simulink model "mars_uav_simulink"  (R2021a)
settings: Solver=ode45  StartTime=0.0  StopTime=30  RelTol=1e-3  EnableMultiTasking=on
undefined symbols (not defined in the file or in its folder): Quad, sigbuilder_block
settings Model: Creator=test  LastModifiedBy=aakash
settings SolverCC: AlgebraicLoopSolver=TrustRegion
settings DataIOCC: SaveFormat=Array  SignalLoggingSaveFormat=ModelDataLogs  ReturnWorkspaceOutputs=off
settings OptimizationCC: ExpressionDepthLimit=2147483647  LifeSpan=inf
settings DebuggingCC: UnderspecifiedInitializationDetection=Classic  MergeDetectMultiDrivingBlocksExec=none  SolverPrmCheckMsg=warning  FcnCallInpInsideContextMsg=warning  StateNameClashWarn=warning  SFUnexpectedBacktrackingDiag=warning  SFNoUnconditionalDefaultTransitionDiag=warning  SFExecutionAtInitializationDiag=none  SFMachineParentedDataDiag=warning  ArithmeticOperatorsInVariantConditions=warning
settings HardwareCC: ProdBitPerPointer=32  ProdBitPerSizeT=32  ProdBitPerPtrDiffT=32  ProdLargestAtomicFloat=None  ProdIntDivRoundTo=Undefined  ProdEndianess=Unspecified  ProdWordSize=32  ProdHWDeviceType=32-bit Generic
settings ModelReferenceCC: PropagateSignalLabelsOutOfModel=off
settings SFSimCC: SimUseLocalCustomCode=off  CustomCodeUndefinedFunction=UseInterfaceOnly
settings RTWCC: RTWUseLocalCustomCode=off
settings CodeAppCC: StateflowObjectComments=on
settings GRTTargetCC: TargetLangStandard=C89/C90 (ANSI)  CombineOutputUpdateFcns=off  GRTInterface=on
settings ConfigComp: CovMetricSettings=dw  CovSaveCumulativeToWorkspaceVar=on  CovSaveSingleToWorkspaceVar=on

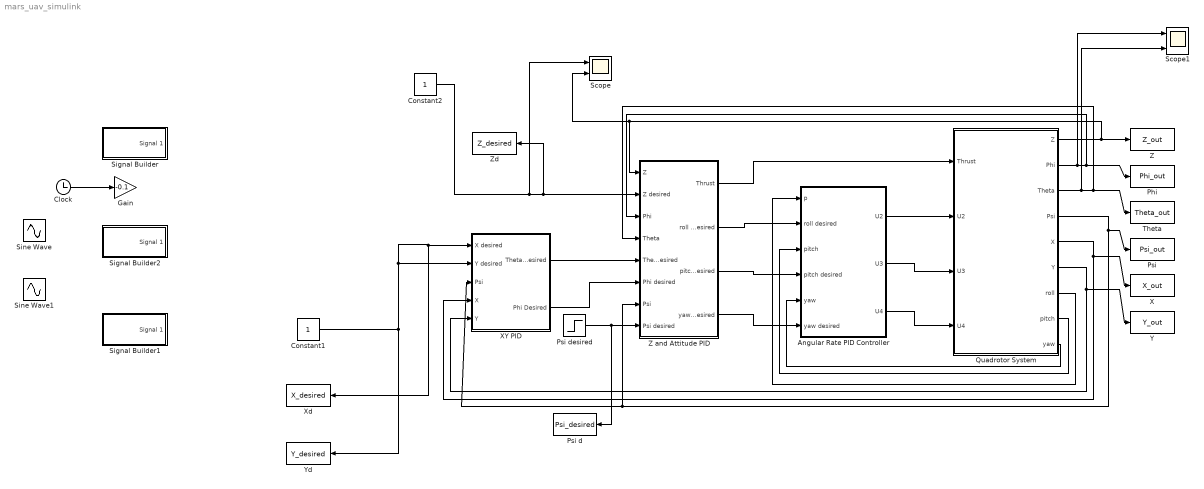
== system mars_uav_simulink ==
  Angular Rate PID Controller : Subsystem
  Clock : Clock
  Constant1 : Constant
  Constant2 : Constant
  Gain : Gain  Gain=-0.1
  Phi : ToWorkspace  VariableName=Phi_out  SaveFormat=Structure  SampleTime=-1
  Psi : ToWorkspace  VariableName=Psi_out  SaveFormat=Structure  SampleTime=-1
  Psi d : ToWorkspace  VariableName=Psi_desired  SaveFormat=Structure  SampleTime=-1
  Psi desired : Step  After=0  SampleTime=0
  Quadrotor System : Subsystem
  Scope : Scope  NumInputPorts=2
  Scope1 : Scope  NumInputPorts=2
  Signal Builder : Subsystem  Tag=STV Subsys  LoadFcn=sigbuilder_block('load');  StartFcn=sigbuilder_block('start');  StopFcn=sigbuilder_block('stop');  ClipboardFcn=sigbuilder_block('clipboard');  mask(Sigbuilder block){tuvar=[0:10]}
      mask help: Simulink:masks:SigbuilderBlock_MD
      mask init:
      | if ~strcmp(get_param(bdroot(gcbh),'SimulationStatus'),'stopped') tuvar = sigbuilder_block('maskInit'); end
      settings: CopyFcn=sigbuilder_block('copy');  DeleteFcn=sigbuilder_block('delete');  ModelCloseFcn=sigbuilder_block('modelClose');  PreSaveFcn=sigbuilder_block('preSave');  PauseFcn=sigbuilder_block('pause');  ContinueFcn=sigbuilder_block('continue');  NameChangeFcn=sigbuilder_block('namechange');  OpenFcn=sigbuilder_block('open',[437.6 199.2 550.4 400 ]);  CloseFcn=sigbuilder_block('close');
      mask Display: plot(0, 0, 100, 100,[2, 2, 32, 32, 2], [68, 8, 8, 68, 68],[32, 2], [38, 38], [32, 19, 2],[53, 60, 44], [32, 17, 17, 2],[16, 16, 31, 31]);txt = getActiveGroup(gcbh);text(2, 100, txt,'verticalAlignment', 'top');
  Signal Builder1 : Subsystem  Tag=STV Subsys  LoadFcn=sigbuilder_block('load');  StartFcn=sigbuilder_block('start');  StopFcn=sigbuilder_block('stop');  ClipboardFcn=sigbuilder_block('clipboard');  mask(Sigbuilder block){tuvar=[0:10]}
      mask help: Simulink:masks:SigbuilderBlock_MD
      mask init:
      | if ~strcmp(get_param(bdroot(gcbh),'SimulationStatus'),'stopped') tuvar = sigbuilder_block('maskInit'); end
      settings: CopyFcn=sigbuilder_block('copy');  DeleteFcn=sigbuilder_block('delete');  ModelCloseFcn=sigbuilder_block('modelClose');  PreSaveFcn=sigbuilder_block('preSave');  PauseFcn=sigbuilder_block('pause');  ContinueFcn=sigbuilder_block('continue');  NameChangeFcn=sigbuilder_block('namechange');  OpenFcn=sigbuilder_block('open',[437.6 199.2 550.4 400 ]);  CloseFcn=sigbuilder_block('close');
      mask Display: plot(0, 0, 100, 100,[2, 2, 32, 32, 2], [68, 8, 8, 68, 68],[32, 2], [38, 38], [32, 19, 2],[53, 60, 44], [32, 17, 17, 2],[16, 16, 31, 31]);txt = getActiveGroup(gcbh);text(2, 100, txt,'verticalAlignment', 'top');
  Signal Builder2 : Subsystem  Tag=STV Subsys  LoadFcn=sigbuilder_block('load');  StartFcn=sigbuilder_block('start');  StopFcn=sigbuilder_block('stop');  ClipboardFcn=sigbuilder_block('clipboard');  mask(Sigbuilder block){tuvar=[0:10]}
      mask help: Simulink:masks:SigbuilderBlock_MD
      mask init:
      | if ~strcmp(get_param(bdroot(gcbh),'SimulationStatus'),'stopped') tuvar = sigbuilder_block('maskInit'); end
      settings: CopyFcn=sigbuilder_block('copy');  DeleteFcn=sigbuilder_block('delete');  ModelCloseFcn=sigbuilder_block('modelClose');  PreSaveFcn=sigbuilder_block('preSave');  PauseFcn=sigbuilder_block('pause');  ContinueFcn=sigbuilder_block('continue');  NameChangeFcn=sigbuilder_block('namechange');  OpenFcn=sigbuilder_block('open',[437.6 199.2 550.4 400 ]);  CloseFcn=sigbuilder_block('close');
      mask Display: plot(0, 0, 100, 100,[2, 2, 32, 32, 2], [68, 8, 8, 68, 68],[32, 2], [38, 38], [32, 19, 2],[53, 60, 44], [32, 17, 17, 2],[16, 16, 31, 31]);txt = getActiveGroup(gcbh);text(2, 100, txt,'verticalAlignment', 'top');
  Sine Wave : Sin  Bias=-1  Frequency=0.1*pi  Phase=pi/2  SampleTime=0
  Sine Wave1 : Sin  Frequency=0.1*pi  SampleTime=0
  Theta : ToWorkspace  VariableName=Theta_out  SaveFormat=Structure  SampleTime=-1
  X : ToWorkspace  VariableName=X_out  SaveFormat=Structure  SampleTime=-1
  XY PID : Subsystem
  Xd : ToWorkspace  VariableName=X_desired  SaveFormat=Structure  SampleTime=-1
  Y : ToWorkspace  VariableName=Y_out  SaveFormat=Structure  SampleTime=-1
  Yd : ToWorkspace  VariableName=Y_desired  SaveFormat=Structure  SampleTime=-1
  Z : ToWorkspace  VariableName=Z_out  SaveFormat=Structure  SampleTime=-1
  Z and Attitude PID : Subsystem
  Zd : ToWorkspace  VariableName=Z_desired  SaveFormat=Structure  SampleTime=-1
  wires:
  Quadrotor System/2(Phi) -> Scope1/1, Phi/1, Z and Attitude PID/3(Phi)
  Quadrotor System/3(Theta) -> Scope1/2, Z and Attitude PID/4(Theta), Theta/1
  Quadrotor System/4(Psi) -> Psi/1, XY PID/3(Psi), Z and Attitude PID/7(Psi)
  Quadrotor System/5(X) -> X/1, XY PID/4(X)
  Quadrotor System/6(Y) -> Y/1, XY PID/5(Y)
  Quadrotor System/1(Z) -> Scope/2, Z and Attitude PID/1(Z), Z/1
  Psi desired/1 -> Z and Attitude PID/8(Psi desired), Psi d/1
  Constant1/1 -> XY PID/1(X desired), Xd/1, XY PID/2(Y desired), Yd/1
  Z and Attitude PID/1(Thrust) -> Quadrotor System/1(Thrust)
  XY PID/2(Phi Desired) -> Z and Attitude PID/6(Phi desired)
  Z and Attitude PID/2(roll desired) -> Angular Rate PID Controller/2(roll desired)
  Z and Attitude PID/3(pitch desired) -> Angular Rate PID Controller/4(pitch desired)
  Z and Attitude PID/4(yaw desired) -> Angular Rate PID Controller/6(yaw desired)
  Quadrotor System/9(yaw) -> Angular Rate PID Controller/5(yaw)
  Quadrotor System/8(pitch) -> Angular Rate PID Controller/3(pitch)
  Quadrotor System/7(roll) -> Angular Rate PID Controller/1(p)
  Angular Rate PID Controller/3(U4) -> Quadrotor System/4(U4)
  Angular Rate PID Controller/2(U3) -> Quadrotor System/3(U3)
  Angular Rate PID Controller/1(U2) -> Quadrotor System/2(U2)
  Clock/1 -> Gain/1
  XY PID/1(Theta Desired) -> Z and Attitude PID/5(Theta desired)
  Constant2/1 -> Scope/1, Zd/1, Z and Attitude PID/2(Z desired)

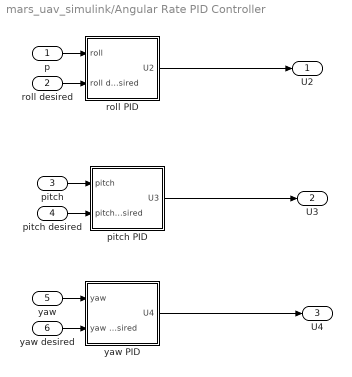
== system mars_uav_simulink/Angular Rate PID Controller ==
  p : Inport
  roll desired : Inport  Port=2
  pitch : Inport  Port=3
  pitch desired : Inport  Port=4
  yaw : Inport  Port=5
  yaw desired : Inport  Port=6
  pitch PID : Subsystem
  roll PID : Subsystem
  yaw PID : Subsystem
  U2 : Outport
  U3 : Outport  Port=2
  U4 : Outport  Port=3
  wires:
  roll PID/1(U2) -> U2/1
  pitch PID/1(U3) -> U3/1
  yaw PID/1(U4) -> U4/1
  p/1 -> roll PID/1(roll)
  roll desired/1 -> roll PID/2(roll desired)
  pitch/1 -> pitch PID/1(pitch)
  pitch desired/1 -> pitch PID/2(pitch desired)
  yaw/1 -> yaw PID/1(yaw)
  yaw desired/1 -> yaw PID/2(yaw desired)

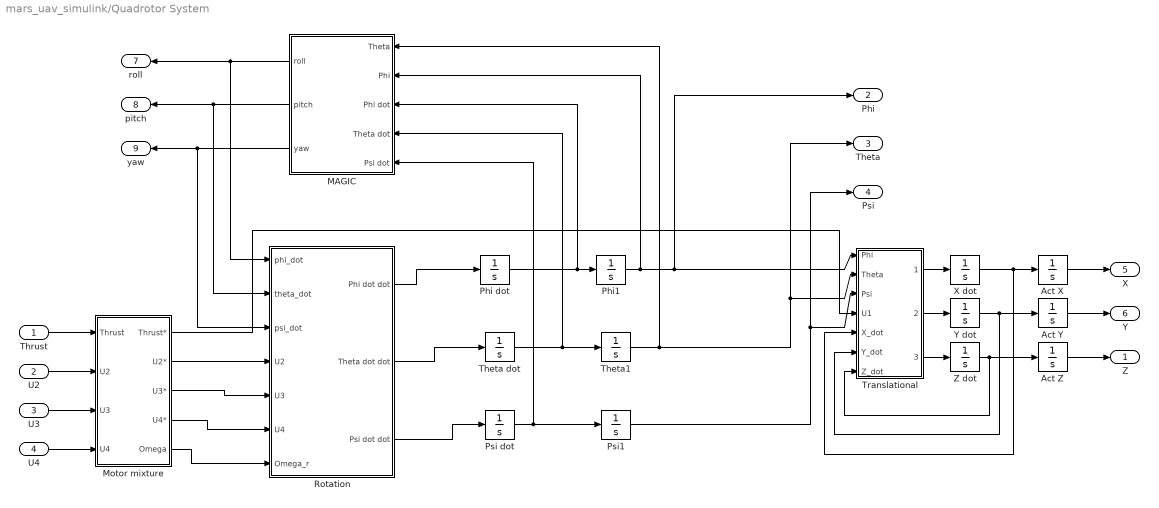
== system mars_uav_simulink/Quadrotor System ==
  Thrust : Inport
  U2 : Inport  Port=2
  U3 : Inport  Port=3
  U4 : Inport  Port=4
  Act X : Integrator
  Act Y : Integrator
  Act Z : Integrator
  "MAGIC " : Subsystem
  Motor mixture : Subsystem
  Phi dot : Integrator
  Phi1 : Integrator  ZeroCross=off
  Psi dot : Integrator  ZeroCross=off
  Psi1 : Integrator  ZeroCross=off
  "Rotation " : Subsystem
  Theta dot : Integrator  ZeroCross=off
  Theta1 : Integrator  ZeroCross=off
  Translational : Subsystem
  X dot : Integrator
  Y dot : Integrator
  Z dot : Integrator
  Z : Outport
  Phi : Outport  Port=2
  Theta : Outport  Port=3
  Psi : Outport  Port=4
  X : Outport  Port=5
  Y : Outport  Port=6
  roll : Outport  Port=7
  pitch : Outport  Port=8
  yaw : Outport  Port=9
  wires:
  "Rotation "/2(Theta dot dot) -> Theta dot/1
  Motor mixture/5(Omega) -> "Rotation "/7(Omega_r)
  Phi1/1 -> Translational/1(Phi), Phi/1, "MAGIC "/2(Phi)
  Theta1/1 -> Translational/2(Theta), Theta/1, "MAGIC "/1(Theta)
  Psi1/1 -> Translational/3(Psi), Psi/1
  Translational/1(X_dot_dot) -> X dot/1
  X dot/1 -> Act X/1, Translational/5(X_dot)
  Y dot/1 -> Act Y/1, Translational/6(Y_dot)
  Translational/2(Y_dot_dot) -> Y dot/1
  Z dot/1 -> Translational/7(Z_dot), Act Z/1
  Translational/3(Z_dot_dot) -> Z dot/1
  Act X/1 -> X/1
  Act Y/1 -> Y/1
  Act Z/1 -> Z/1
  Psi dot/1 -> Psi1/1, "MAGIC "/5(Psi dot)
  Theta dot/1 -> Theta1/1, "MAGIC "/4(Theta dot)
  Phi dot/1 -> Phi1/1, "MAGIC "/3(Phi dot)
  "Rotation "/3(Psi dot dot) -> Psi dot/1
  "Rotation "/1(Phi dot dot) -> Phi dot/1
  U4/1 -> Motor mixture/4(U4)
  U2/1 -> Motor mixture/2(U2)
  U3/1 -> Motor mixture/3(U3)
  Motor mixture/2(U2*) -> "Rotation "/4(U2)
  Motor mixture/3(U3*) -> "Rotation "/5(U3)
  Motor mixture/1(Thrust*) -> Translational/4(U1)
  Motor mixture/4(U4*) -> "Rotation "/6(U4)
  "MAGIC "/1(roll) -> roll/1, "Rotation "/1(phi_dot)
  "MAGIC "/2(pitch) -> pitch/1, "Rotation "/2(theta_dot)
  "MAGIC "/3(yaw) -> yaw/1, "Rotation "/3(psi_dot)
  Thrust/1 -> Motor mixture/1(Thrust)

== system mars_uav_simulink/Signal Builder ==
  Demux : Demux  Tag=STV Demux  Outputs=1
      settings: DisplayOption=none
  FromWs : FromWorkspace  Tag=STV FromWs  VariableName=tuvar
      SigBuilderData=|
      | common.afterFinalStr = 'Extrapolate'
      | common.sampleTime = 0
      | dataSet.timeRange = [0 30]
      | dataSet.name = 'Group 1'
      | sbobj.Groups.Name = 'Group 1'
      | sbobj.Groups.Signals.Name = 'Signal 1'
      | sbobj.Groups.Signals.XData = [0 5 10 20 25 30]
      | sbobj.Groups.Signals.YData = [0 1 1 -1 -1 0]
      | sbobj.Groups.TimeRange = [0 30]
  Signal 1 : Outport  Tag=STV Outport
  wires:
  Demux/1 -> Signal 1/1
  FromWs/1 -> Demux/1

== system mars_uav_simulink/Signal Builder1 ==
  Demux : Demux  Tag=STV Demux  Outputs=1
      settings: DisplayOption=none
  FromWs : FromWorkspace  Tag=STV FromWs  VariableName=tuvar
      SigBuilderData=|
      | common.afterFinalStr = 'Extrapolate'
      | common.sampleTime = 0
      | dataSet.timeRange = [0 30]
      | dataSet.name = 'Group 1'
      | sbobj.Groups.Name = 'Group 1'
      | sbobj.Groups.Signals.Name = 'Signal 1'
      | sbobj.Groups.Signals.XData = [0 4 6 30]
      | sbobj.Groups.Signals.YData = [0 0 0 0]
      | sbobj.Groups.TimeRange = [0 30]
  Signal 1 : Outport  Tag=STV Outport
  wires:
  Demux/1 -> Signal 1/1
  FromWs/1 -> Demux/1

== system mars_uav_simulink/Signal Builder2 ==
  Demux : Demux  Tag=STV Demux  Outputs=1
      settings: DisplayOption=none
  FromWs : FromWorkspace  Tag=STV FromWs  VariableName=tuvar
      SigBuilderData=|
      | common.afterFinalStr = 'Extrapolate'
      | common.sampleTime = 0
      | dataSet.timeRange = [0 30]
      | dataSet.name = 'Group 1'
      | sbobj.Groups.Name = 'Group 1'
      | sbobj.Groups.Signals.Name = 'Signal 1'
      | sbobj.Groups.Signals.XData = [0 5 10 20 25 30]
      | sbobj.Groups.Signals.YData = [0 0 1 1 0 0]
      | sbobj.Groups.TimeRange = [0 30]
  Signal 1 : Outport  Tag=STV Outport
  wires:
  Demux/1 -> Signal 1/1
  FromWs/1 -> Demux/1

== system mars_uav_simulink/XY PID ==
  X desired : Inport
  Y desired : Inport  Port=2
  Psi : Inport  Port=3
  X : Inport  Port=4
  Y : Inport  Port=5
  Actual Position GF to BF : Subsystem
  Desired Position GF to BF : Subsystem
  X PID : Subsystem
  Y PID : Subsystem
  Theta Desired : Outport
  Phi Desired : Outport  Port=2
  wires:
  X PID/1(Theta Desired) -> Theta Desired/1
  Y PID/1(Phi Desired) -> Phi Desired/1
  X desired/1 -> Desired Position GF to BF/1(X GF)
  Y desired/1 -> Desired Position GF to BF/2(Y GF)
  Desired Position GF to BF/1("X Bf ") -> X PID/1(X desired)
  Desired Position GF to BF/2(Y Bf) -> Y PID/1(Y desired)
  X/1 -> Actual Position GF to BF/1(X GF)
  Y/1 -> Actual Position GF to BF/2(Y GF)
  Actual Position GF to BF/1("X Bf ") -> X PID/2(X)
  Actual Position GF to BF/2(Y Bf) -> Y PID/2(Y)
  Psi/1 -> Desired Position GF to BF/3(Psi), Actual Position GF to BF/3(Psi)

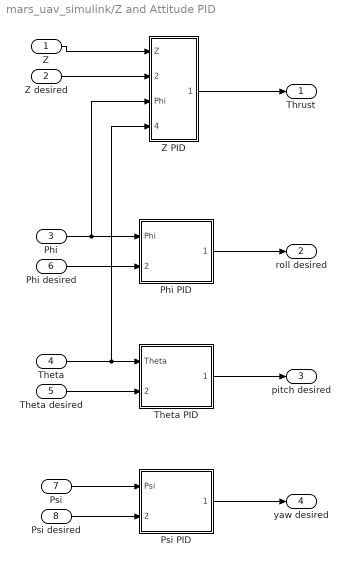
== system mars_uav_simulink/Z and Attitude PID ==
  Z : Inport
  Z desired : Inport  Port=2
  Phi : Inport  Port=3
  Theta : Inport  Port=4
  Theta desired : Inport  Port=5
  Phi desired : Inport  Port=6
  Psi : Inport  Port=7
  Psi desired : Inport  Port=8
  Phi PID : Subsystem
  Psi PID : Subsystem
  Theta PID : Subsystem
  Z PID : Subsystem
  Thrust : Outport
  roll desired : Outport  Port=2
  pitch desired : Outport  Port=3
  yaw desired : Outport  Port=4
  wires:
  Z PID/1(Thrust) -> Thrust/1
  Z desired/1 -> Z PID/2(Z desired)
  Z/1 -> Z PID/1(Z)
  Phi desired/1 -> Phi PID/2(Phi desired)
  Phi/1 -> Phi PID/1(Phi), Z PID/3(Phi)
  Psi desired/1 -> Psi PID/2(Psi desired)
  Psi/1 -> Psi PID/1(Psi)
  Theta desired/1 -> Theta PID/2(Theta desired)
  Theta/1 -> Theta PID/1(Theta), Z PID/4(Theta)
  Phi PID/1(roll rate desired) -> roll desired/1
  Psi PID/1(yaw rate desired) -> yaw desired/1
  Theta PID/1(pitch rate desired) -> pitch desired/1

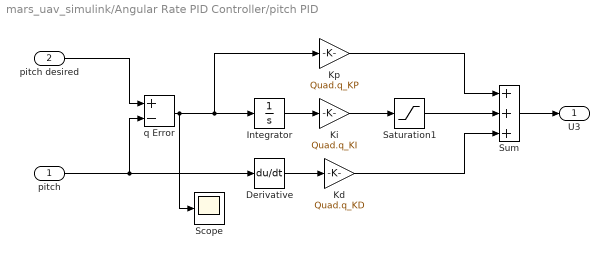
== system mars_uav_simulink/Angular Rate PID Controller/pitch PID ==
  pitch : Inport
  pitch desired : Inport  Port=2
  Derivative : Derivative
  Integrator : Integrator
  Kd : Gain  Gain=Quad.q_KD
  Ki : Gain  Gain=Quad.q_KI
  Kp : Gain  Gain=Quad.q_KP
  Saturation1 : Saturate  UpperLimit=Quad.U3_max  LowerLimit=Quad.U3_min
  Scope : Scope
  Sum : Sum  Inputs=+++
  q Error : Sum  Inputs=+-
  U3 : Outport
  wires:
  pitch/1 -> q Error/2, Derivative/1
  pitch desired/1 -> q Error/1
  Derivative/1 -> Kd/1
  Kp/1 -> Sum/1
  Sum/1 -> U3/1
  q Error/1 -> Integrator/1, Kp/1, Scope/1
  Integrator/1 -> Ki/1
  Kd/1 -> Sum/3
  Ki/1 -> Saturation1/1
  Saturation1/1 -> Sum/2

== system mars_uav_simulink/Angular Rate PID Controller/roll PID ==
  roll : Inport
  roll desired : Inport  Port=2
  Derivative : Derivative
  Integrator : Integrator
  Kd : Gain  Gain=Quad.p_KD
  Ki : Gain  Gain=Quad.p_KI
  Kp : Gain  Gain=Quad.p_KP
  Psi Error : Sum  Inputs=+-
  Saturation1 : Saturate  UpperLimit=Quad.U2_max  LowerLimit=Quad.U2_min
  Sum : Sum  Inputs=+++
  U2 : Outport
  wires:
  roll/1 -> Psi Error/2, Derivative/1
  roll desired/1 -> Psi Error/1
  Derivative/1 -> Kd/1
  Kp/1 -> Sum/1
  Sum/1 -> U2/1
  Psi Error/1 -> Integrator/1, Kp/1
  Integrator/1 -> Ki/1
  Kd/1 -> Sum/3
  Ki/1 -> Saturation1/1
  Saturation1/1 -> Sum/2

== system mars_uav_simulink/Angular Rate PID Controller/yaw PID ==
  yaw : Inport
  yaw desired : Inport  Port=2
  Derivative : Derivative
  Kd : Gain  Gain=Quad.r_KD
  Kp : Gain  Gain=Quad.r_KP
  Psi Error : Sum  Inputs=+-
  Sum : Sum
  U4 : Outport
  wires:
  yaw/1 -> Psi Error/2, Derivative/1
  yaw desired/1 -> Psi Error/1
  Derivative/1 -> Kd/1
  Kp/1 -> Sum/1
  Sum/1 -> U4/1
  Psi Error/1 -> Kp/1
  Kd/1 -> Sum/2

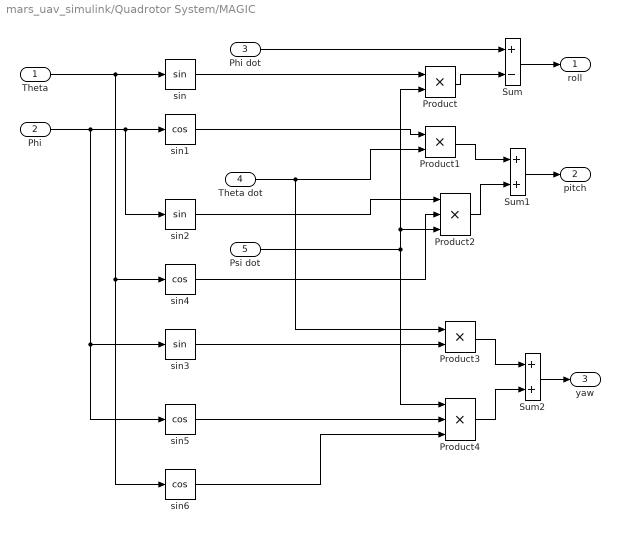
== system mars_uav_simulink/Quadrotor System/MAGIC  ==
  Theta : Inport
  Phi : Inport  Port=2
  Phi dot : Inport  Port=3
  Theta dot : Inport  Port=4
  Psi dot : Inport  Port=5
  Product : Product  RndMeth=Zero
  Product1 : Product  RndMeth=Zero
  Product2 : Product  Inputs=3  RndMeth=Zero
  Product3 : Product  RndMeth=Zero
  Product4 : Product  Inputs=3  RndMeth=Zero
  Sum : Sum  Inputs=+-
  Sum1 : Sum
  Sum2 : Sum
  sin : Trigonometry
  sin{1,4..6} (4 alike) : Trigonometry  Operator=cos
  sin2 : Trigonometry
  sin3 : Trigonometry
  roll : Outport
  pitch : Outport  Port=2
  yaw : Outport  Port=3
  wires:
  Phi dot/1 -> Sum/1
  Theta/1 -> sin4/1, sin6/1, sin/1
  sin/1 -> Product/1
  Psi dot/1 -> Product/2, Product2/3, Product4/1
  Product/1 -> Sum/2
  Sum/1 -> roll/1
  Phi/1 -> sin1/1, sin2/1, sin3/1, sin5/1
  sin1/1 -> Product1/1
  Theta dot/1 -> Product1/2, Product3/1
  Product1/1 -> Sum1/1
  sin2/1 -> Product2/1
  sin4/1 -> Product2/2
  Product2/1 -> Sum1/2
  Sum1/1 -> pitch/1
  sin3/1 -> Product3/2
  sin5/1 -> Product4/2
  sin6/1 -> Product4/3
  Product3/1 -> Sum2/1
  Product4/1 -> Sum2/2
  Sum2/1 -> yaw/1

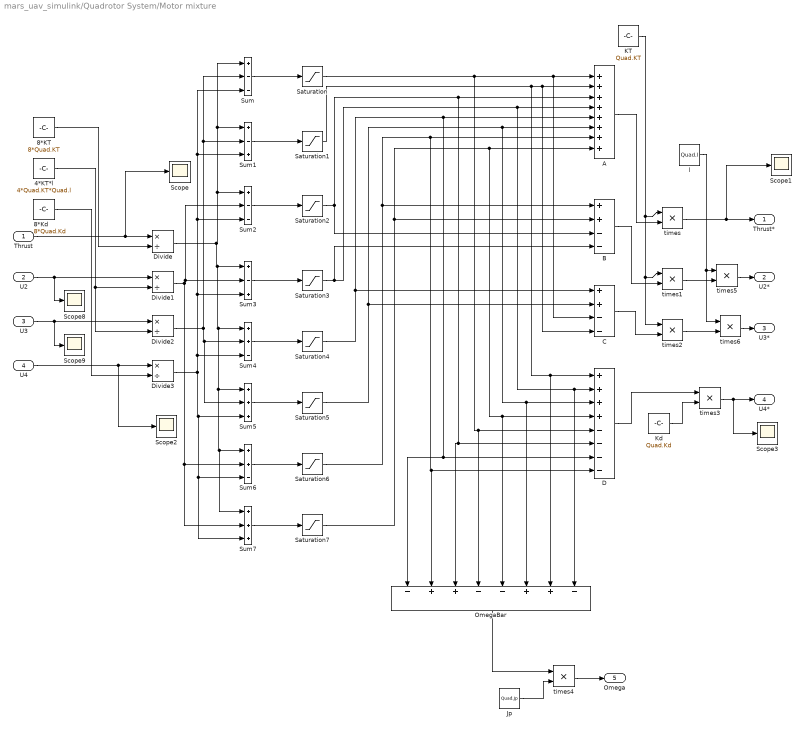
== system mars_uav_simulink/Quadrotor System/Motor mixture ==
  Thrust : Inport
  U2 : Inport  Port=2
  U3 : Inport  Port=3
  U4 : Inport  Port=4
  4*KT*l : Constant  Value=4*Quad.KT*Quad.l
  8*KT : Constant  Value=8*Quad.KT
  8*Kd : Constant  Value=8*Quad.Kd
  A : Sum  Inputs=++++++++
  B : Sum  Inputs=++--
  C : Sum  Inputs=++--
  D : Sum  Inputs=++++----
  Divide{,1..3} (4 alike) : Product  Inputs=*/
  Jp : Constant  Value=Quad.Jp
  KT : Constant  Value=Quad.KT
  Kd : Constant  Value=Quad.Kd
  OmegaBar : Sum  Inputs=-++--++-
  Saturation{,1..7} (8 alike) : Saturate  UpperLimit=Quad.max_motor_speed^2  LowerLimit=Quad.min_motor_speed^2  ZeroCross=off
  Scope{,1..3,8..9} (6 alike) : Scope
  Sum : Sum  Inputs=+--
  Sum1 : Sum  Inputs=+-+
  Sum2 : Sum  Inputs=+--
  Sum3 : Sum  Inputs=+-+
  Sum4 : Sum  Inputs=++-
  Sum5 : Sum  Inputs=+++
  Sum6 : Sum  Inputs=++-
  Sum7 : Sum  Inputs=+++
  l : Constant  Value=Quad.l
  times{,1..6} (7 alike) : Product  Inputs=**
  Thrust* : Outport
  U2* : Outport  Port=2
  U3* : Outport  Port=3
  U4* : Outport  Port=4
  Omega : Outport  Port=5
  wires:
  Thrust/1 -> Divide/1, Scope/1
  8*KT/1 -> Divide/2
  U2/1 -> Divide1/1, Scope8/1
  4*KT*l/1 -> Divide1/2, Divide2/2
  U3/1 -> Divide2/1, Scope9/1
  U4/1 -> Divide3/1, Scope2/1
  8*Kd/1 -> Divide3/2
  OmegaBar/1 -> times4/1
  times4/1 -> Omega/1
  KT/1 -> times/1, times1/1, times2/1
  A/1 -> times/2
  B/1 -> times1/2
  C/1 -> times2/2
  D/1 -> times3/1
  Kd/1 -> times3/2
  times/1 -> Thrust*/1, Scope1/1
  times3/1 -> U4*/1, Scope3/1
  Jp/1 -> times4/2
  times5/1 -> U2*/1
  times6/1 -> U3*/1
  l/1 -> times5/1, times6/1
  times1/1 -> times5/2
  times2/1 -> times6/2
  Divide/1 -> Sum7/1, Sum6/1, Sum5/1, Sum4/1, Sum3/1, Sum1/1, Sum/1, Sum2/1
  Divide2/1 -> Sum5/2, Sum4/2, Sum1/2, Sum/2
  Divide3/1 -> Sum7/3, Sum6/3, Sum5/3, Sum4/3, Sum3/3, Sum2/3, Sum1/3, Sum/3
  Divide1/1 -> Sum7/2, Sum6/2, Sum3/2, Sum2/2
  Sum/1 -> Saturation/1
  Sum1/1 -> Saturation1/1
  Sum2/1 -> Saturation2/1
  Sum3/1 -> Saturation3/1
  Sum4/1 -> Saturation4/1
  Sum5/1 -> Saturation5/1
  Sum6/1 -> Saturation6/1
  Sum7/1 -> Saturation7/1
  Saturation/1 -> D/5, OmegaBar/4, C/3, A/1
  Saturation1/1 -> D/1, OmegaBar/7, A/2, C/4
  Saturation2/1 -> B/3, D/6, OmegaBar/3, A/3
  Saturation3/1 -> OmegaBar/8, D/2, A/4, B/4
  Saturation4/1 -> OmegaBar/1, D/7, A/5, C/1
  Saturation5/1 -> C/2, D/3, OmegaBar/6, A/6
  Saturation6/1 -> D/8, OmegaBar/2, A/7, B/1
  Saturation7/1 -> B/2, D/4, OmegaBar/5, A/8

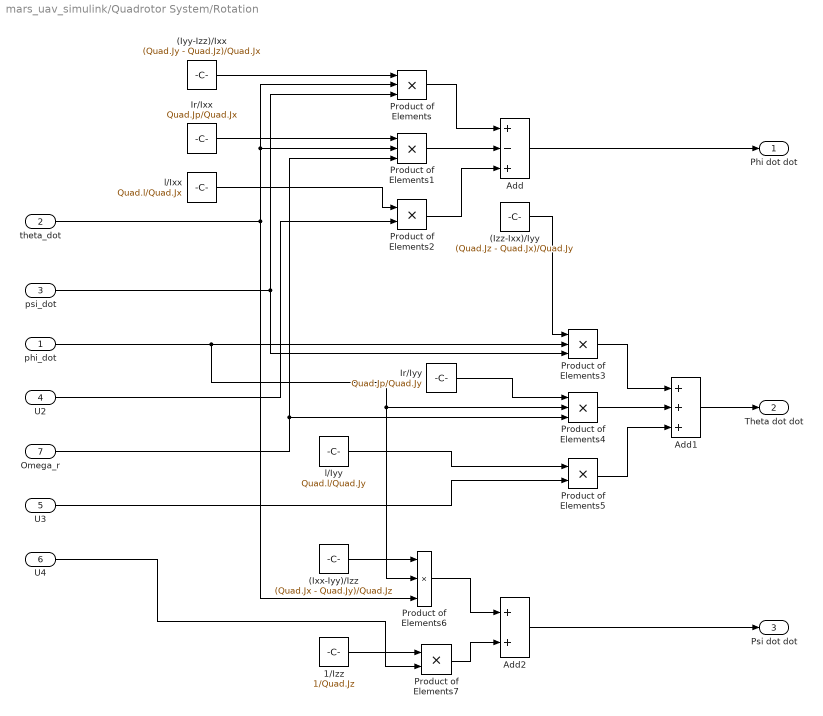
== system mars_uav_simulink/Quadrotor System/Rotation  ==
  phi_dot : Inport
  theta_dot : Inport  Port=2
  psi_dot : Inport  Port=3
  U2 : Inport  Port=4
  U3 : Inport  Port=5
  U4 : Inport  Port=6
  Omega_r : Inport  Port=7
  (Ixx-Iyy)/Izz : Constant  Value=(Quad.Jx - Quad.Jy)/Quad.Jz
  (Iyy-Izz)/Ixx : Constant  Value=(Quad.Jy - Quad.Jz)/Quad.Jx
  (Izz-Ixx)/Iyy : Constant  Value=(Quad.Jz - Quad.Jx)/Quad.Jy
  1/Izz : Constant  Value=1/Quad.Jz
  Add : Sum  Inputs=+-+
  Add1 : Sum  Inputs=+++
  Add2 : Sum
  Ir/Ixx : Constant  Value=Quad.Jp/Quad.Jx
  Ir/Iyy : Constant  Value=Quad.Jp/Quad.Jy
  Product of Elements{,1,3..4,6} (5 alike) : Product  Inputs=3
  Product of Elements2 : Product
  Product of Elements5 : Product
  Product of Elements7 : Product
  l/Ixx : Constant  Value=Quad.l/Quad.Jx
  l/Iyy : Constant  Value=Quad.l/Quad.Jy
  Phi dot dot : Outport
  Theta dot dot : Outport  Port=2
  Psi dot dot : Outport  Port=3
  wires:
  Product of Elements/1 -> Add/1
  Product of Elements1/1 -> Add/2
  Product of Elements2/1 -> Add/3
  Add/1 -> Phi dot dot/1
  (Iyy-Izz)/Ixx/1 -> Product of Elements/1
  theta_dot/1 -> Product of Elements6/3, Product of Elements/2, Product of Elements1/2
  psi_dot/1 -> Product of Elements3/3, Product of Elements/3
  Ir/Ixx/1 -> Product of Elements1/1
  l/Ixx/1 -> Product of Elements2/1
  U2/1 -> Product of Elements2/2
  Omega_r/1 -> Product of Elements1/3, Product of Elements4/3
  Product of Elements3/1 -> Add1/1
  Product of Elements4/1 -> Add1/2
  Product of Elements5/1 -> Add1/3
  Add1/1 -> Theta dot dot/1
  (Izz-Ixx)/Iyy/1 -> Product of Elements3/1
  Ir/Iyy/1 -> Product of Elements4/1
  l/Iyy/1 -> Product of Elements5/1
  U3/1 -> Product of Elements5/2
  phi_dot/1 -> Product of Elements4/2, Product of Elements6/2, Product of Elements3/2
  Product of Elements7/1 -> Add2/2
  Add2/1 -> Psi dot dot/1
  U4/1 -> Product of Elements7/2
  1/Izz/1 -> Product of Elements7/1
  (Ixx-Iyy)/Izz/1 -> Product of Elements6/1
  Product of Elements6/1 -> Add2/1

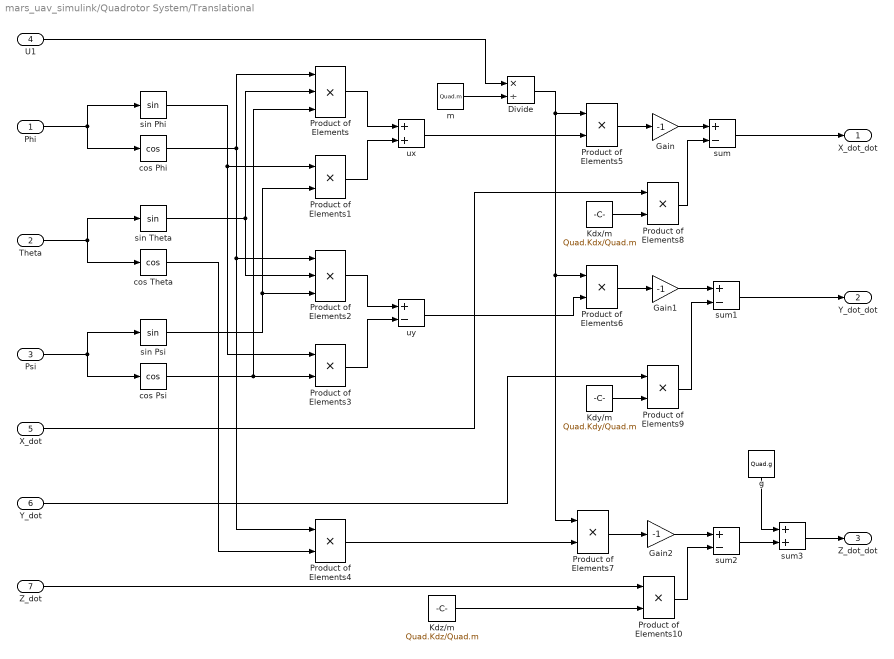
== system mars_uav_simulink/Quadrotor System/Translational ==
  Phi : Inport
  Theta : Inport  Port=2
  Psi : Inport  Port=3
  U1 : Inport  Port=4
  X_dot : Inport  Port=5
  Y_dot : Inport  Port=6
  Z_dot : Inport  Port=7
  Divide : Product  Inputs=*/
  Gain : Gain  Gain=-1
  Gain1 : Gain  Gain=-1
  Gain2 : Gain  Gain=-1
  Kdx/m : Constant  Value=Quad.Kdx/Quad.m
  Kdy/m : Constant  Value=Quad.Kdy/Quad.m
  Kdz/m : Constant  Value=Quad.Kdz/Quad.m
  Product of Elements : Product  Inputs=3
  Product of Elements{1,3..10} (9 alike) : Product
  Product of Elements2 : Product  Inputs=3
  cos Phi : Trigonometry  Operator=cos
  cos Psi : Trigonometry  Operator=cos
  cos Theta : Trigonometry  Operator=cos
  g : Constant  Value=Quad.g
  m : Constant  Value=Quad.m
  sin Phi : Trigonometry
  sin Psi : Trigonometry
  sin Theta : Trigonometry
  sum : Sum  Inputs=+-
  sum1 : Sum  Inputs=+-
  sum2 : Sum  Inputs=+-
  sum3 : Sum
  ux : Sum
  uy : Sum  Inputs=+-
  X_dot_dot : Outport
  Y_dot_dot : Outport  Port=2
  Z_dot_dot : Outport  Port=3
  wires:
  Phi/1 -> sin Phi/1, cos Phi/1
  Theta/1 -> sin Theta/1, cos Theta/1
  Psi/1 -> sin Psi/1, cos Psi/1
  sin Theta/1 -> Product of Elements/2, Product of Elements2/2
  cos Psi/1 -> Product of Elements/3, Product of Elements3/2
  cos Phi/1 -> Product of Elements/1, Product of Elements2/1, Product of Elements4/1
  sin Phi/1 -> Product of Elements1/1, Product of Elements3/1
  sin Psi/1 -> Product of Elements1/2, Product of Elements2/3
  Product of Elements/1 -> ux/1
  Product of Elements1/1 -> ux/2
  ux/1 -> Product of Elements5/2
  Product of Elements2/1 -> uy/1
  Product of Elements3/1 -> uy/2
  uy/1 -> Product of Elements6/2
  cos Theta/1 -> Product of Elements4/2
  Product of Elements4/1 -> Product of Elements7/2
  U1/1 -> Divide/1
  m/1 -> Divide/2
  Divide/1 -> Product of Elements5/1, Product of Elements6/1, Product of Elements7/1
  sum3/1 -> Z_dot_dot/1
  Product of Elements5/1 -> Gain/1
  Product of Elements6/1 -> Gain1/1
  X_dot/1 -> Product of Elements8/1
  Kdx/m/1 -> Product of Elements8/2
  Gain/1 -> sum/1
  Product of Elements8/1 -> sum/2
  sum/1 -> X_dot_dot/1
  Y_dot/1 -> Product of Elements9/1
  Kdy/m/1 -> Product of Elements9/2
  Gain1/1 -> sum1/1
  Product of Elements9/1 -> sum1/2
  sum1/1 -> Y_dot_dot/1
  Z_dot/1 -> Product of Elements10/1
  Kdz/m/1 -> Product of Elements10/2
  Product of Elements7/1 -> Gain2/1
  g/1 -> sum3/1
  sum2/1 -> sum3/2
  Product of Elements10/1 -> sum2/2
  Gain2/1 -> sum2/1

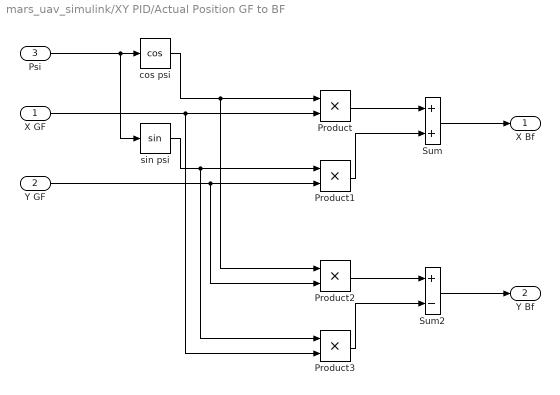
== system mars_uav_simulink/XY PID/Actual Position GF to BF ==
  X GF : Inport
  Y GF : Inport  Port=2
  Psi : Inport  Port=3
  Product{,1..3} (4 alike) : Product  RndMeth=Zero
  Sum : Sum
  Sum2 : Sum  Inputs=+-
  cos psi : Trigonometry  Operator=cos
  sin psi : Trigonometry
  "X Bf " : Outport
  Y Bf : Outport  Port=2
  wires:
  Psi/1 -> cos psi/1, sin psi/1
  cos psi/1 -> Product/1, Product2/1
  X GF/1 -> Product/2, Product3/2
  Product/1 -> Sum/1
  sin psi/1 -> Product1/1, Product3/1
  Y GF/1 -> Product1/2, Product2/2
  Product1/1 -> Sum/2
  Sum/1 -> "X Bf "/1
  Product2/1 -> Sum2/1
  Product3/1 -> Sum2/2
  Sum2/1 -> Y Bf/1

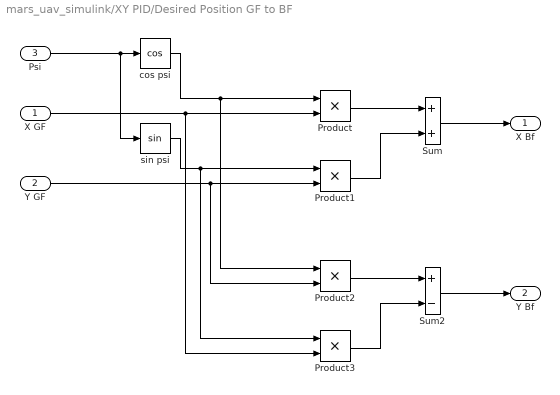
== system mars_uav_simulink/XY PID/Desired Position GF to BF ==
  X GF : Inport
  Y GF : Inport  Port=2
  Psi : Inport  Port=3
  Product{,1..3} (4 alike) : Product  RndMeth=Zero
  Sum : Sum
  Sum2 : Sum  Inputs=+-
  cos psi : Trigonometry  Operator=cos
  sin psi : Trigonometry
  "X Bf " : Outport
  Y Bf : Outport  Port=2
  wires:
  Psi/1 -> cos psi/1, sin psi/1
  cos psi/1 -> Product/1, Product2/1
  X GF/1 -> Product/2, Product3/2
  Product/1 -> Sum/1
  sin psi/1 -> Product1/1, Product3/1
  Y GF/1 -> Product1/2, Product2/2
  Product1/1 -> Sum/2
  Sum/1 -> "X Bf "/1
  Product2/1 -> Sum2/1
  Product3/1 -> Sum2/2
  Sum2/1 -> Y Bf/1

== system mars_uav_simulink/XY PID/X PID ==
  X desired : Inport
  X : Inport  Port=2
  Derivative : Derivative
  Integrator : Integrator
  Kd : Gain  Gain=Quad.X_KD
  Ki : Gain  Gain=Quad.X_KI
  Kp : Gain  Gain=Quad.X_KP
  Saturation1 : Saturate  UpperLimit=Quad.theta_max  LowerLimit=-Quad.theta_max
  Saturation2 : Saturate  UpperLimit=Quad.theta_max  LowerLimit=-Quad.theta_max
  Sum : Sum  Inputs=---
  X Error : Sum  Inputs=+-
  Theta Desired : Outport
  wires:
  X/1 -> X Error/2, Derivative/1
  X desired/1 -> X Error/1
  Derivative/1 -> Kd/1
  Kp/1 -> Sum/1
  Sum/1 -> Saturation2/1
  X Error/1 -> Integrator/1, Kp/1
  Integrator/1 -> Ki/1
  Kd/1 -> Sum/3
  Saturation2/1 -> Theta Desired/1
  Ki/1 -> Saturation1/1
  Saturation1/1 -> Sum/2

== system mars_uav_simulink/XY PID/Y PID ==
  Y desired : Inport
  Y : Inport  Port=2
  Derivative : Derivative
  Integrator : Integrator
  Kd : Gain  Gain=Quad.Y_KD
  Ki : Gain  Gain=Quad.Y_KI
  Kp : Gain  Gain=Quad.Y_KP
  Saturation1 : Saturate  UpperLimit=Quad.phi_max  LowerLimit=-Quad.phi_max
  Saturation2 : Saturate  UpperLimit=Quad.phi_max  LowerLimit=-Quad.phi_max
  Sum : Sum  Inputs=+++
  Y Error : Sum  Inputs=+-
  Phi Desired : Outport
  wires:
  Y/1 -> Y Error/2, Derivative/1
  Y desired/1 -> Y Error/1
  Derivative/1 -> Kd/1
  Kp/1 -> Sum/1
  Sum/1 -> Saturation2/1
  Y Error/1 -> Integrator/1, Kp/1
  Integrator/1 -> Ki/1
  Kd/1 -> Sum/3
  Ki/1 -> Saturation1/1
  Saturation1/1 -> Sum/2
  Saturation2/1 -> Phi Desired/1

== system mars_uav_simulink/Z and Attitude PID/Phi PID ==
  Phi : Inport
  Phi desired : Inport  Port=2
  Derivative : Derivative
  Kd : Gain  Gain=Quad.phi_KD
  Kp : Gain  Gain=Quad.phi_KP
  Phi Error : Sum  Inputs=+-
  Sum : Sum
  roll rate desired : Outport
  wires:
  Phi/1 -> Phi Error/2, Derivative/1
  Phi desired/1 -> Phi Error/1
  Derivative/1 -> Kd/1
  Kp/1 -> Sum/1
  Sum/1 -> roll rate desired/1
  Phi Error/1 -> Kp/1
  Kd/1 -> Sum/2

== system mars_uav_simulink/Z and Attitude PID/Psi PID ==
  Psi : Inport
  Psi desired : Inport  Port=2
  Derivative : Derivative
  Kd : Gain  Gain=Quad.psi_KD
  Kp : Gain  Gain=Quad.psi_KP
  Psi Error : Sum  Inputs=+-
  Sum : Sum
  yaw rate desired : Outport
  wires:
  Psi/1 -> Psi Error/2, Derivative/1
  Psi desired/1 -> Psi Error/1
  Derivative/1 -> Kd/1
  Kp/1 -> Sum/1
  Sum/1 -> yaw rate desired/1
  Psi Error/1 -> Kp/1
  Kd/1 -> Sum/2

== system mars_uav_simulink/Z and Attitude PID/Theta PID ==
  Theta : Inport
  Theta desired : Inport  Port=2
  Derivative : Derivative
  Kd : Gain  Gain=Quad.theta_KD
  Kp : Gain  Gain=Quad.theta_KP
  Sum : Sum
  Theta Error : Sum  Inputs=+-
  pitch rate desired : Outport
  wires:
  Theta/1 -> Derivative/1, Theta Error/2
  Theta desired/1 -> Theta Error/1
  Derivative/1 -> Kd/1
  Kp/1 -> Sum/1
  Sum/1 -> pitch rate desired/1
  Theta Error/1 -> Kp/1
  Kd/1 -> Sum/2

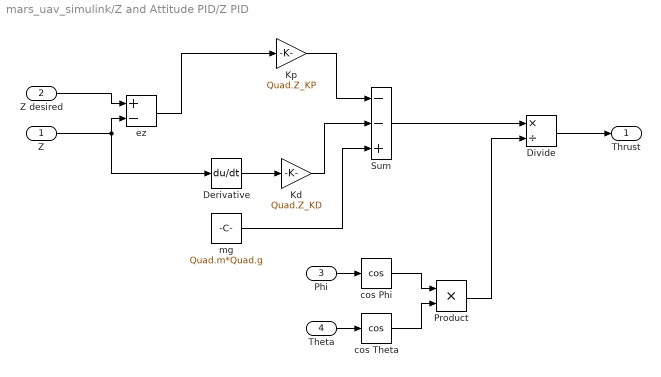
== system mars_uav_simulink/Z and Attitude PID/Z PID ==
  Z : Inport
  Z desired : Inport  Port=2
  Phi : Inport  Port=3
  Theta : Inport  Port=4
  Derivative : Derivative
  Divide : Product  Inputs=*/
  Kd : Gain  Gain=Quad.Z_KD
  Kp : Gain  Gain=Quad.Z_KP
  Product : Product  RndMeth=Zero
  Sum : Sum  Inputs=--+
  cos Phi : Trigonometry  Operator=cos
  cos Theta : Trigonometry  Operator=cos
  ez : Sum  Inputs=+-
  mg : Constant  Value=Quad.m*Quad.g
  Thrust : Outport
  wires:
  Z desired/1 -> ez/1
  cos Phi/1 -> Product/1
  cos Theta/1 -> Product/2
  Product/1 -> Divide/2
  Phi/1 -> cos Phi/1
  Theta/1 -> cos Theta/1
  Z/1 -> ez/2, Derivative/1
  Derivative/1 -> Kd/1
  Kp/1 -> Sum/1
  ez/1 -> Kp/1
  Sum/1 -> Divide/1
  Divide/1 -> Thrust/1
  mg/1 -> Sum/3
  Kd/1 -> Sum/2
